simulink model "pro_simu"  (R2020b)
settings: Solver=VariableStepAuto  StartTime=0.0  StopTime=3.5  RelTol=1e-3
values from neighbouring files (symbols this model uses):
  A = subs(Jx,[x1,x2,x3,x4],[0,0,0,0])    [linearisation.m]    (also in pro_main_code.m = [0 1 0 0;0 -15.47 41.68 0;0 0 0 1;0 -14.89 84.05 0])
  B = subs(Ju,u,0)    [linearisation.m]    (also in pro_main_code.m = [0;27.12;0;23.13])
  C = [1 0 0 0]    [pro_main_code.m]
  Gcl0_inv = inv(Gcl0)    [pro_main_code.m]
  K_11 = K_acker1(1,1:4)    [pro_main_code.m]
  K_11_lqr = K_lqr1(1,1:4)    [pro_main_code.m]
  K_12 = K_acker1(1,5)    [pro_main_code.m]
  K_12_lqr = K_lqr1(1,5)    [pro_main_code.m]
  K_acker = acker(A,B,des_pole)    [pro_main_code.m]
libraries: simulink x4
settings Model: Creator=Benyamin (hamireZ)  LastModifiedBy=Benyamin (hamireZ)

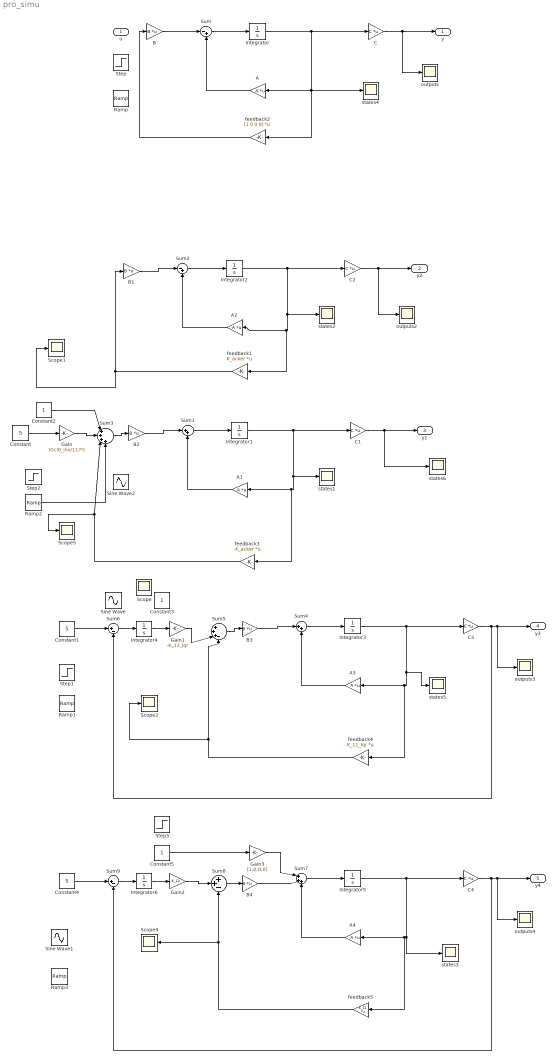
== system pro_simu ==
  u : Inport
  A{,1..4} (5 alike) : Gain  Gain=A  Multiplication=Matrix(K*u) (u vector)
  B{,1..4} (5 alike) : Gain  Gain=B  Multiplication=Matrix(K*u) (u vector)
  C{,1..4} (5 alike) : Gain  Gain=C  Multiplication=Matrix(K*u) (u vector)
  Constant : Constant  Value=5
  Constant1 : Constant  Value=5
  Constant2 : Constant
  Constant3 : Constant
  Constant4 : Constant  Value=5
  Constant5 : Constant
  Gain : Gain  Gain=(Gcl0_inv/11)*5
  Gain1 : Gain  Gain=-K_12_lqr
  Gain2 : Gain  Gain=-K_12
  Gain3 : Gain  Gain=[1;0;0;0]
  Integrator{,1..3,5} (5 alike) : Integrator  InitialCondition=[0;0;1;0]
  Integrator4 : Integrator
  Integrator6 : Integrator
  Ramp : simulink/Sources/Ramp  slope=1  start=0  InitialOutput=0
  Ramp1 : simulink/Sources/Ramp  slope=0.5  start=0  InitialOutput=0
  Ramp2 : simulink/Sources/Ramp  slope=0.5  start=0  InitialOutput=0
  Ramp3 : simulink/Sources/Ramp  slope=1  start=0  InitialOutput=0
  Scope{,1..2,4..5} (5 alike) : Scope
  Sine Wave : Sin  Amplitude=-10  Frequency=10  SampleTime=0
  Sine Wave1 : Sin  Amplitude=-1  Frequency=2  SampleTime=0
  Sine Wave2 : Sin  SampleTime=0
  Step : Step  Before=1  After=0  SampleTime=0
  Step1 : Step  Time=2  SampleTime=0
  Step2 : Step  Time=2  SampleTime=0
  Step3 : Step  Before=1  After=0  SampleTime=0
  Sum : Sum  Inputs=|-+
  Sum1 : Sum  Inputs=|++
  Sum2 : Sum  Inputs=|-+
  Sum3 : Sum  Inputs=|++++
  Sum4 : Sum  Inputs=|++
  Sum5 : Sum  Inputs=|+++-
  Sum6 : Sum  Inputs=|+-
  Sum7 : Sum  Inputs=|+++
  Sum8 : Sum  Inputs=++-
  Sum9 : Sum  Inputs=|+-
  feedback1 : Gain  Gain=K_acker  Multiplication=Matrix(K*u) (u vector)
  feedback2 : Gain  Gain=[1 0 0 0]  Multiplication=Matrix(K*u) (u vector)
  feedback3 : Gain  Gain=-K_acker  Multiplication=Matrix(K*u) (u vector)
  feedback4 : Gain  Gain=K_11_lqr  Multiplication=Matrix(K*u) (u vector)
  feedback5 : Gain  Gain=K_11  Multiplication=Matrix(K*u) (u vector)
  outputs{,2..4} (4 alike) : Scope
  states{1..6} (6 alike) : Scope
  y : Outport
  y2 : Outport  Port=2
  y1 : Outport  Port=3
  y3 : Outport  Port=4
  y4 : Outport  Port=5
  wires:
  C/1 -> outputs/1, y/1
  Sum/1 -> Integrator/1
  A/1 -> Sum/2
  C2/1 -> outputs2/1, y2/1
  Sum2/1 -> Integrator2/1
  A2/1 -> Sum2/2
  Integrator2/1 -> feedback1/1, A2/1, states2/1, C2/1
  B/1 -> Sum/1
  B2/1 -> Sum1/1
  Integrator1/1 -> C1/1, states1/1, A1/1, feedback3/1
  A1/1 -> Sum1/2
  Sum1/1 -> Integrator1/1
  C1/1 -> states6/1, y1/1
  feedback3/1 -> Scope5/1, Sum3/3
  Sum3/1 -> B2/1
  Sum5/1 -> B3/1
  feedback4/1 -> Scope2/1, Sum5/4
  C3/1 -> Sum6/2, outputs3/1, y3/1
  Sum4/1 -> Integrator3/1
  A3/1 -> Sum4/2
  Integrator3/1 -> feedback4/1, A3/1, states5/1, C3/1
  B3/1 -> Sum4/1
  Integrator4/1 -> Gain1/1
  Sum6/1 -> Integrator4/1
  Constant1/1 -> Sum6/1
  Constant/1 -> Gain/1
  Gain/1 -> Sum3/2
  Gain1/1 -> Sum5/3
  B4/1 -> Sum7/2
  Integrator5/1 -> C4/1, states3/1, A4/1, feedback5/1
  A4/1 -> Sum7/3
  Sum7/1 -> Integrator5/1
  C4/1 -> y4/1, outputs4/1, Sum9/2
  feedback5/1 -> Scope4/1, Sum8/3
  Sum8/1 -> B4/1
  Gain2/1 -> Sum8/2
  feedback1/1 -> Scope1/1, B1/1
  B1/1 -> Sum2/1
  Integrator/1 -> feedback2/1, states4/1, A/1, C/1
  feedback2/1 -> B/1
  Constant2/1 -> Sum3/1
  Ramp2/1 -> Sum3/4
  Sum9/1 -> Integrator6/1
  Integrator6/1 -> Gain2/1
  Constant4/1 -> Sum9/1
  Constant5/1 -> Gain3/1
  Gain3/1 -> Sum7/1
